simulink model "THD"  (R2021b)
settings: Solver=VariableStepAuto  StartTime=0.0  StopTime=0.2  MaxStep=1e-4  RelTol=1e-3
libraries: spsMosfetLib x4, spsMultimeterLib x3, spsACVoltageSourceLib x2, spsSeriesRLCBranchLib x2, spsThyristorLib x2, spspowerguiLib x1
settings Model: Creator=Dong  LastModifiedBy=Dong

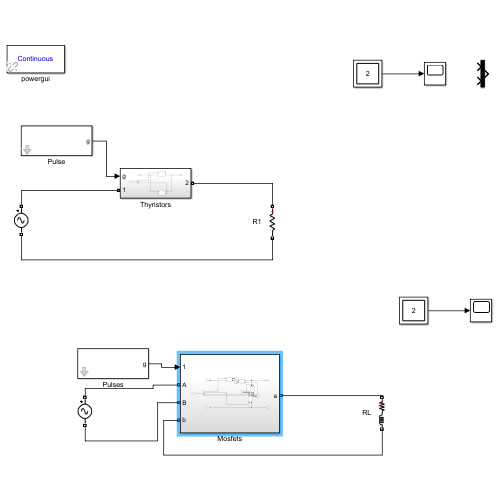
[thumbnail: Simulink's stored preview of the top-level diagram]
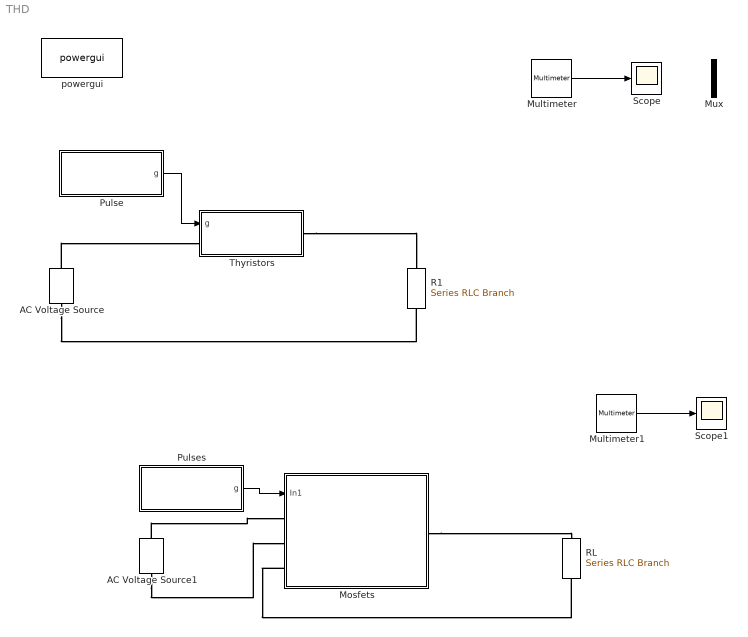
== system THD ==
  AC Voltage Source : spsACVoltageSourceLib/AC Voltage Source  Amplitude=100  Phase=0  Frequency=50  SampleTime=0  Measurements=None  BusType=swing  Pref=10e3  Qref=0  Qmin=-inf  Qmax=+inf
  AC Voltage Source1 : spsACVoltageSourceLib/AC Voltage Source  Amplitude=100  Phase=0  Frequency=50  SampleTime=0  Measurements=Voltage  BusType=swing  Pref=10e3  Qref=0  Qmin=-inf  Qmax=+inf
  Mosfets : Subsystem
  Multimeter : spsMultimeterLib/Multimeter  PhasorSimulation=off  OutputType=Complex  sel=[1 4]  L=5  Gain=[1 1]  yselected={'Ub: R1','Ib: R1'};  PSBOutputType=1  PSBequivalent=0  AxesSetting=[0,0.1,-100,100]  Display=0  SavedBlockNames=-11
  Multimeter1 : spsMultimeterLib/Multimeter  PhasorSimulation=off  OutputType=Complex  sel=[2 5]  L=5  Gain=[1 1]  yselected={'Ub: RL','Ib: RL'};  PSBOutputType=1  PSBequivalent=0  AxesSetting=[0,0.1,-100,100]  Display=0  SavedBlockNames=-11
  Mux : Mux  Inputs=2
  Pulse : Subsystem  mask{alpha=30, frez=50}
      mask prompts: alpha "Phasewinkel"; frez "Frequenz"
  Pulses : Subsystem  mask{alpha=30, frez=50}
      mask prompts: alpha "Phasewinkel"; frez "Frequenz"
  R1 : spsSeriesRLCBranchLib/Series RLC Branch  LConnTagsString=__new0  RConnTagsString=__new0  BranchType=R  Resistance=8  Inductance=1e-3  SetiL0=off  InitialCurrent=0  Capacitance=1e-6  Setx0=off  InitialVoltage=0  Measurements=Branch voltage and current
  RL : spsSeriesRLCBranchLib/Series RLC Branch  LConnTagsString=__new0  RConnTagsString=__new0  BranchType=RL  Resistance=8  Inductance=10e-3  SetiL0=off  InitialCurrent=0  Capacitance=1e-6  Setx0=off  InitialVoltage=0  Measurements=Branch voltage and current
  Scope : Scope
  Scope1 : Scope
  Thyristors : Subsystem
  powergui : spspowerguiLib/powergui  Priority=1  SimulationMode=Continuous  SampleTime=50e-6  frequency=60  Iterations=50  frequencyindice=50  Pbase=100e6  ErrMax=1e-4  UnitsV=kV  UnitsW=MW  buscounter=0  FunctionMessages=off  echomessages=off  EnableUseOfTLC=off  CurrentSourceSwitches=off  DisableSnubberDevices=off  DisableRonSwitches=off  DisableVfSwitches=off  DisplayEquations=off  AutomaticDiscreteSolvers=off  SolverType=Tustin/Backward Euler (TBE)  Interpol=off  ExternalGateDelay=off  methode=off  Ts=100  x0status=blocks  SPID=on  SwTol=0  HookPort=off  NonlinearTolerance=1e-4  nMaxIteration=100  ContinueOnMaxIteration=off  RestoreLinks=warning  ResistiveCurrentMeasurement=off  Frange=[0:2:500]  Ylog=off  Xlog=on  ShowGrid=off  save=off  variable=ZData  structure=0  ZoomFFT=off  StartTime=0.0  cycles=1  DisplayStyle=1  fundamental=60  FreqAxis=off  MaxFrequency=1000  frequencyindicesteady=1  RmsSteady=1  display=off
  wires:
  Multimeter/1 -> Scope/1
  Pulse/1(g) -> Thyristors/1(g)
  Multimeter1/1 -> Scope1/1
  Pulses/1(g) -> Mosfets/1(In1)
  connections:
  AC Voltage Source/LConn1 -- R1/RConn1
  AC Voltage Source/RConn1 -- Thyristors/LConn1
  Thyristors/RConn1 -- R1/LConn1
  AC Voltage Source1/RConn1 -- Mosfets/LConn1
  AC Voltage Source1/LConn1 -- Mosfets/LConn2
  Mosfets/RConn1 -- RL/LConn1
  Mosfets/LConn3 -- RL/RConn1

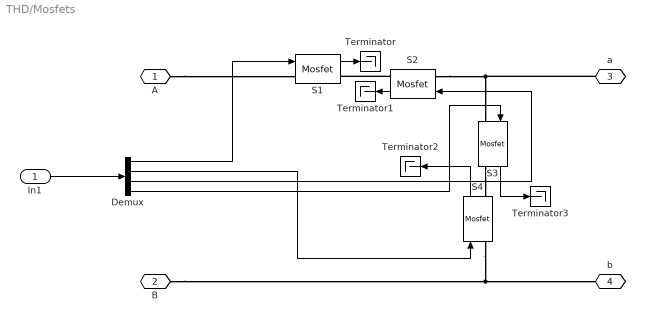
== system THD/Mosfets ==
  In1 : Inport
  Demux : Demux
  S{1..4} (4 alike) : spsMosfetLib/Mosfet  Ron=0.1  Lon=0  Rd=0.01  Vfd=0  IC=0  Rs=1e5  Cs=inf  Measurements=on
  Terminator{,1..3} (4 alike) : Terminator
  A : PMIOPort  Side=Left
  B : PMIOPort  Port=2  Side=Left
  a : PMIOPort  Port=3  Side=Right
  b : PMIOPort  Port=4  Side=Left
  wires:
  In1/1 -> Demux/1
  Demux/1 -> S1/1
  Demux/2 -> S4/1
  Demux/3 -> S2/1
  Demux/4 -> S3/1
  S1/1 -> Terminator/1
  S2/1 -> Terminator1/1
  S4/1 -> Terminator2/1
  S3/1 -> Terminator3/1
  connections:
  S2/RConn1 -- S1/RConn1
  S3/RConn1 -- S4/RConn1
  S2/LConn1 -- a/RConn1 -- S3/LConn1
  S4/LConn1 -- B/RConn1 -- b/RConn1
  A/RConn1 -- S1/LConn1

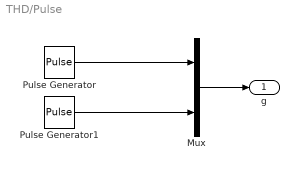
== system THD/Pulse ==
  Mux : Mux  Inputs=2
  Pulse Generator : DiscretePulseGenerator  PulseType=Time based  Period=1/frez  PulseWidth=5  PhaseDelay=(alpha/360)*(1/frez)
  Pulse Generator1 : DiscretePulseGenerator  PulseType=Time based  Period=1/frez  PulseWidth=5  PhaseDelay=(alpha+180/360)*(1/frez)
  g : Outport
  wires:
  Pulse Generator/1 -> Mux/1
  Pulse Generator1/1 -> Mux/2
  Mux/1 -> g/1

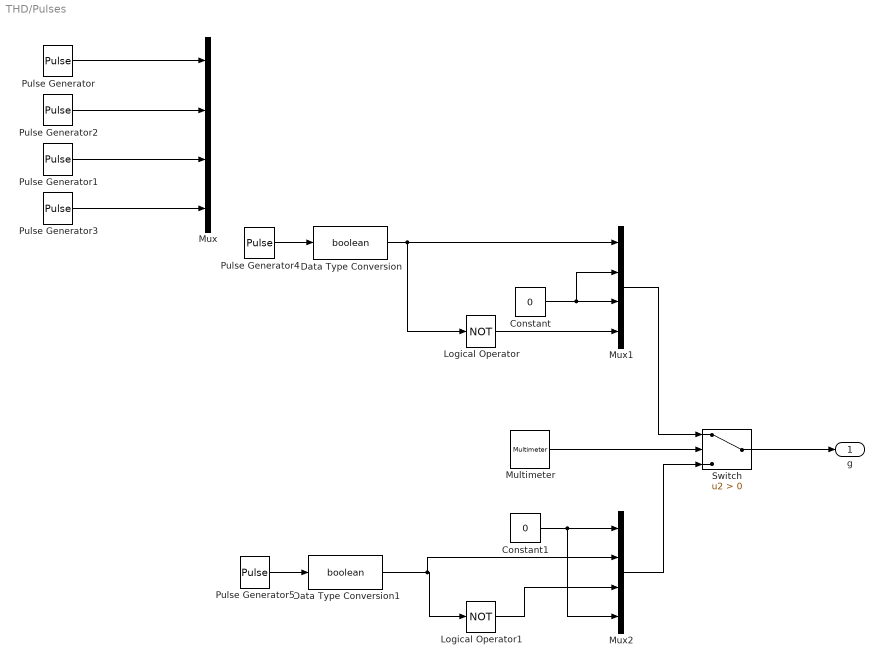
== system THD/Pulses ==
  Constant : Constant  Value=0  OutDataTypeStr=boolean
  Constant1 : Constant  Value=0  OutDataTypeStr=boolean
  Data Type Conversion : DataTypeConversion  OutDataTypeStr=boolean
  Data Type Conversion1 : DataTypeConversion  OutDataTypeStr=boolean
  Logical Operator : Logic  Operator=NOT  AllPortsSameDT=off  OutDataTypeStr=boolean
  Logical Operator1 : Logic  Operator=NOT  AllPortsSameDT=off  OutDataTypeStr=boolean
  Multimeter : spsMultimeterLib/Multimeter  PhasorSimulation=off  OutputType=Complex  sel=3  L=5  Gain=1  yselected={'Usrc: AC Voltage Source1'};  PSBOutputType=1  PSBequivalent=0  AxesSetting=[0,0.1,-100,100]  Display=0  SavedBlockNames=-11
  Mux : Mux
  Mux1 : Mux
  Mux2 : Mux
  Pulse Generator : DiscretePulseGenerator  PulseType=Time based  Period=1/frez  PulseWidth=5  PhaseDelay=(alpha+180)/360*(1/frez)
  Pulse Generator1 : DiscretePulseGenerator  PulseType=Time based  Period=1/frez  PulseWidth=5  PhaseDelay=(alpha/360)*(1/frez)
  Pulse Generator2 : DiscretePulseGenerator  PulseType=Time based  Period=1/frez  PulseWidth=5  PhaseDelay=(alpha+180)/360*(1/frez)
  Pulse Generator3 : DiscretePulseGenerator  PulseType=Time based  Period=1/frez  PulseWidth=5  PhaseDelay=(alpha/360)*(1/frez)
  Pulse Generator4 : DiscretePulseGenerator  PulseType=Time based  Period=1/20e3  PulseWidth=50
  Pulse Generator5 : DiscretePulseGenerator  PulseType=Time based  Period=1/20e3  PulseWidth=50
  Switch : Switch  Criteria=u2 > Threshold
  g : Outport
  wires:
  Pulse Generator/1 -> Mux/1
  Pulse Generator2/1 -> Mux/2
  Pulse Generator1/1 -> Mux/3
  Pulse Generator3/1 -> Mux/4
  Switch/1 -> g/1
  Multimeter/1 -> Switch/2
  Mux1/1 -> Switch/1
  Constant/1 -> Mux1/2, Mux1/3
  Pulse Generator4/1 -> Data Type Conversion/1
  Data Type Conversion/1 -> Logical Operator/1, Mux1/1
  Logical Operator/1 -> Mux1/4
  Data Type Conversion1/1 -> Mux2/2, Logical Operator1/1
  Pulse Generator5/1 -> Data Type Conversion1/1
  Mux2/1 -> Switch/3
  Constant1/1 -> Mux2/4, Mux2/1
  Logical Operator1/1 -> Mux2/3

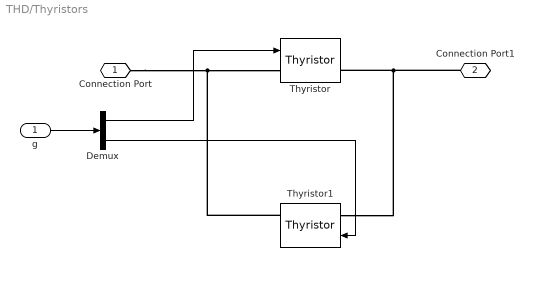
== system THD/Thyristors ==
  g : Inport
  Demux : Demux  Outputs=2
  Thyristor : spsThyristorLib/Thyristor  Ron=0.001  Lon=0  Vf=0.8  IC=0  Rs=500  Cs=250e-9  Measurements=on
  Thyristor1 : spsThyristorLib/Thyristor  Ron=0.001  Lon=0  Vf=0.8  IC=0  Rs=500  Cs=250e-9  Measurements=on
  Connection Port : PMIOPort  Side=Left
  Connection Port1 : PMIOPort  Port=2  Side=Right
  wires:
  g/1 -> Demux/1
  Demux/1 -> Thyristor/1
  Demux/2 -> Thyristor1/1
  connections:
  Connection Port/RConn1 -- Thyristor1/RConn1 -- Thyristor/LConn1
  Connection Port1/RConn1 -- Thyristor1/LConn1 -- Thyristor/RConn1
